simulink model "Intro"  (R2025b)
settings: Solver=VariableStepAuto  StartTime=0.0  StopTime=10  MaxStep=0.01  RelTol=1e-3
settings Model: NumberOfSteps=100  Creator=night  LastModifiedBy=night

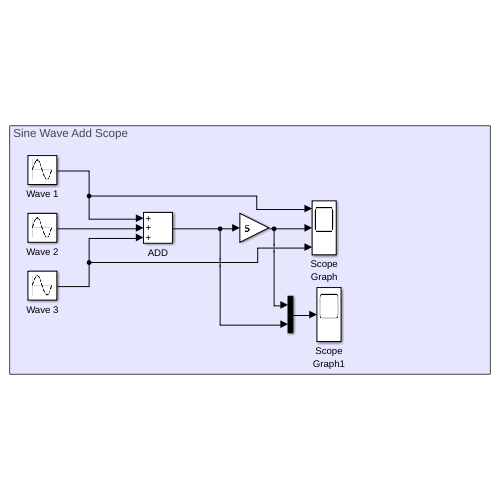
[thumbnail: Simulink's stored preview of the top-level diagram]
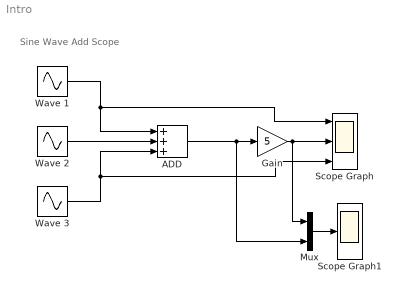
== system Intro ==
  note: Sine Wave Add Scope
  ADD : Sum  Inputs=+++
  Gain : Gain  Gain=5
  Mux : Mux  Inputs=2
  Scope Graph : Scope  NumInputPorts=3
      settings: TimeSpan=10  ActiveDisplayYMinimum=-12.499986958278871  ActiveDisplayYMaximum=12.499959554759947  YLabel=Amptitude
  Scope Graph1 : Scope
      settings: TimeSpan=10  ActiveDisplayYMinimum=-53.218276643963293  ActiveDisplayYMaximum=58.085443563719636  YLabel=Amptitude
  Wave 1 : Sin  Amplitude=10  Frequency=8  SampleTime=0
  Wave 2 : Sin  SampleTime=0
  Wave 3 : Sin  Frequency=10  SampleTime=0
  wires:
  Wave 1/1 -> Scope Graph/1, ADD/1
  Wave 2/1 -> ADD/2
  Wave 3/1 -> Scope Graph/3, ADD/3
  ADD/1 -> Mux/2, Gain/1
  Gain/1 -> Mux/1, Scope Graph/2
  Mux/1 -> Scope Graph1/1
